simulink model "controlled_system"  (R2020b)
settings: Solver=FixedStepAuto  StartTime=0.0  StopTime=10.0  FixedStep=1e-4  RelTol=1e-3
settings Model: Creator=avina  LastModifiedBy=avina

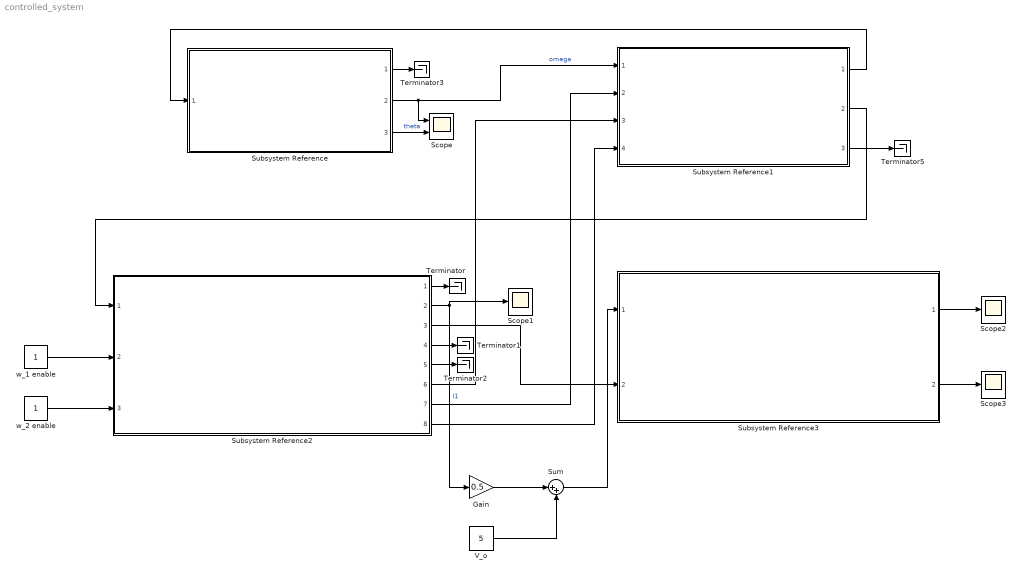
== system controlled_system ==
  Gain : Gain  Gain=0.5
  Scope : Scope  NumInputPorts=2
  Scope1 : Scope
  Scope2 : Scope
  Scope3 : Scope
  Subsystem Reference : Subsystem  ReferencedSubsystem=Pendulum
  Subsystem Reference1 : Subsystem  ReferencedSubsystem=Motor_circuit
  Subsystem Reference2 : Subsystem  ReferencedSubsystem=Tank_system
  Subsystem Reference3 : Subsystem  ReferencedSubsystem=Dissipator_circuit
  Sum : Sum  Inputs=|++
  Terminator{,1..3,5} (5 alike) : Terminator
  V_o : Constant  Value=5
  w_1 enable : Constant
  w_2 enable : Constant
  wires:
  Subsystem Reference/2 -> Scope/1, Subsystem Reference1/1  "omega"
  Subsystem Reference1/1 -> Subsystem Reference/1
  Subsystem Reference1/2 -> Subsystem Reference2/1
  Subsystem Reference2/3 -> Subsystem Reference3/2
  Subsystem Reference2/6 -> Subsystem Reference1/3
  Subsystem Reference2/7 -> Subsystem Reference1/2
  Subsystem Reference2/8 -> Subsystem Reference1/4
  Subsystem Reference2/2 -> Scope1/1, Gain/1  "l1"
  Gain/1 -> Sum/1
  V_o/1 -> Sum/2
  Sum/1 -> Subsystem Reference3/1
  Subsystem Reference2/1 -> Terminator/1
  Subsystem Reference2/5 -> Terminator2/1
  Subsystem Reference2/4 -> Terminator1/1
  Subsystem Reference/1 -> Terminator3/1
  Subsystem Reference1/3 -> Terminator5/1
  Subsystem Reference3/2 -> Scope3/1
  w_1 enable/1 -> Subsystem Reference2/2
  w_2 enable/1 -> Subsystem Reference2/3
  Subsystem Reference/3 -> Scope/2  "theta"
  Subsystem Reference3/1 -> Scope2/1
